simulink model "proj_parachot"  (R2015a)
settings: Solver=ode3  StartTime=0.0  StopTime=3  FixedStep=0.01  RelTol=1e-3
values from neighbouring files (symbols this model uses):
  Bj = 10    [proj_parachotM.m]
  Bp = 100    [proj_parachotM.m]
  Kr = 400    [proj_parachotM.m]
  Mj = 60    [proj_parachotM.m]
  Mp = 10    [proj_parachotM.m]
libraries: fl_lib x15, nesl_utility x7
settings Model: Creator=ahmed alaa  LastModifiedBy=ahmed alaa

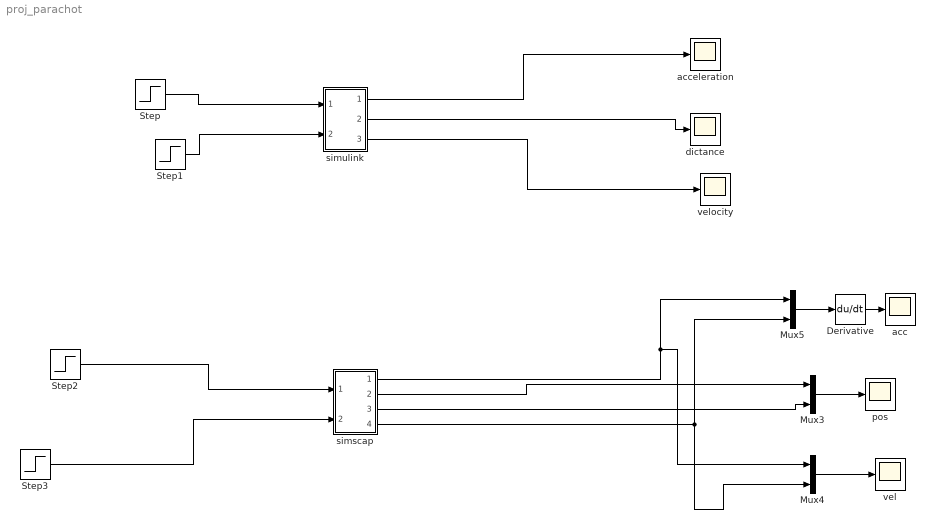
== system proj_parachot ==
  Derivative : Derivative
  Mux3 : Mux  Inputs=2
  Mux4 : Mux  Inputs=2
  Mux5 : Mux  Inputs=2
  Step{,1..3} (4 alike) : Step  Time=0  SampleTime=0
  acc : Scope
      settings: SaveName=ScopeData3
  "acceleration " : Scope
      settings: SaveName=ScopeData2
  dictance : Scope
  pos : Scope
      settings: SaveName=ScopeData4
  simscap : Subsystem
  simulink : Subsystem
  vel : Scope
      settings: SaveName=ScopeData5
  velocity : Scope
  wires:
  Step/1 -> simulink/1(In1)
  Step1/1 -> simulink/2(In2)
  simulink/1(Out1) -> "acceleration "/1
  simulink/2(Out2) -> dictance/1
  simulink/3(Out3) -> velocity/1
  simscap/3(Out3) -> Mux3/2
  simscap/2(Out2) -> Mux3/1
  Step3/1 -> simscap/2(In2)
  Step2/1 -> simscap/1(In1)
  simscap/4(Out4) -> Mux4/2, Mux5/2
  simscap/1(Out1) -> Mux5/1, Mux4/1
  Mux5/1 -> Derivative/1
  Mux3/1 -> pos/1
  Derivative/1 -> acc/1
  Mux4/1 -> vel/1

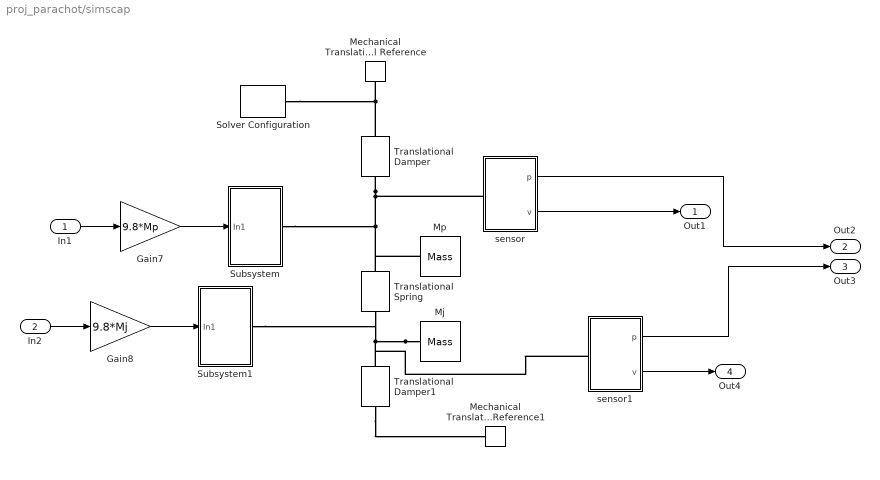
== system proj_parachot/simscap ==
  In1 : Inport
  In2 : Inport  Port=2
  Gain7 : Gain  Gain=9.8*Mp
  Gain8 : Gain  Gain=9.8*Mj
  Mechanical Translational Reference : fl_lib/Mechanical/Translational Elements/Mechanical Translational Reference
  Mechanical Translational Reference1 : fl_lib/Mechanical/Translational Elements/Mechanical Translational Reference
  Mj : fl_lib/Mechanical/Translational Elements/Mass  mass=Mj kg  v_specify=on  v_priority=High  v=20 m/s  f_specify=off  f_priority=High  f=0 N
  Mp : fl_lib/Mechanical/Translational Elements/Mass  mass=Mp kg  v_specify=on  v_priority=High  v=20 m/s  f_specify=off  f_priority=High  f=0 N
  Solver Configuration : nesl_utility/Solver Configuration  PhysicalDomain=network_engine_domain  SubClassName=solver  LeftPortType=input  RightPortType=generic  Accelerate=off  Tones=[]  Harmonics=[]  SimulateNoise=off  Profile=off  UseLocalSampling=off  EnableSwitchedLinearOptims=on  FrequencyDomain=off  UseCCode=off  RelTol=0.001  AbsTol=1e-06  MinStep=1e-09  ToWorkspace=off  RevertToSquareIcSolve=off  NumHomotopyIterations=100  DoDC=off  ResidualTolerance=1e-09  UseLocalSolver=off  LocalSolverChoice=NE_BACKWARD_EULER_ADVANCER  LocalSolverSampleTime=0.001  DoFixedCost=off  MaxNonlinIter=3  MaxModeIter=2  LinearAlgebra=Sparse  DelaysMemoryBudget=1024  AutomaticFiltering=on  FilteringTimeConstant=0.001
  Subsystem : Subsystem
  Subsystem1 : Subsystem
  Translational Damper : fl_lib/Mechanical/Translational Elements/Translational Damper  D=Bp N/(m/s)  v_specify=off  v_priority=High  v=0 m/s  f_specify=off  f_priority=High  f=0 N
  Translational Damper1 : fl_lib/Mechanical/Translational Elements/Translational Damper  D=Bj N/(m/s)  v_specify=off  v_priority=High  v=0 m/s  f_specify=off  f_priority=High  f=0 N
  Translational Spring : fl_lib/Mechanical/Translational Elements/Translational Spring  spr_rate=Kr N/m  v_specify=off  v_priority=High  v=0 m/s  f_specify=off  f_priority=High  f=0 N  x_specify=off  x_priority=High  x=0 m
  sensor : Subsystem
  sensor1 : Subsystem
  Out1 : Outport
  Out2 : Outport  Port=2
  Out3 : Outport  Port=3
  Out4 : Outport  Port=4
  wires:
  Gain7/1 -> Subsystem/1(In1)
  In2/1 -> Gain8/1
  In1/1 -> Gain7/1
  sensor1/1(p) -> Out3/1
  Gain8/1 -> Subsystem1/1(In1)
  sensor/1(p) -> Out2/1
  sensor/2(v) -> Out1/1
  sensor1/2(v) -> Out4/1
  connections:
  Translational Damper1/RConn1 -- Mechanical Translational Reference1/LConn1
  Solver Configuration/RConn1 -- Mechanical Translational Reference/LConn1 -- Translational Damper/LConn1
  Translational Damper/RConn1 -- sensor/LConn1 -- Subsystem/RConn1 -- Translational Spring/LConn1 -- Mp/LConn1
  Mj/LConn1 -- sensor1/LConn1 -- Translational Damper1/LConn1 -- Translational Spring/RConn1 -- Subsystem1/RConn1

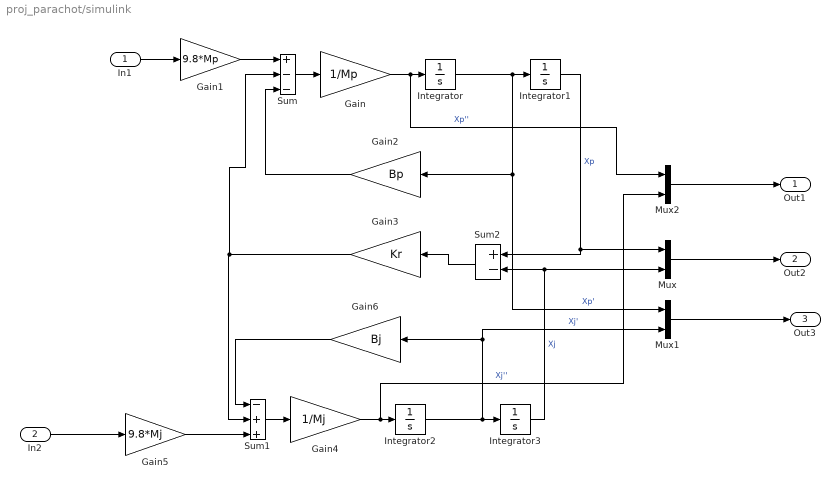
== system proj_parachot/simulink ==
  In1 : Inport
  In2 : Inport  Port=2
  Gain : Gain  Gain=1/Mp
  Gain1 : Gain  Gain=9.8*Mp
  Gain2 : Gain  Gain=Bp
  Gain3 : Gain  Gain=Kr
  Gain4 : Gain  Gain=1/Mj
  Gain5 : Gain  Gain=9.8*Mj
  Gain6 : Gain  Gain=Bj
  Integrator : Integrator  InitialCondition=20
  Integrator1 : Integrator
  Integrator2 : Integrator  InitialCondition=20
  Integrator3 : Integrator
  Mux : Mux  Inputs=2
  Mux1 : Mux  Inputs=2
  Mux2 : Mux  Inputs=2
  Sum : Sum  Inputs=+--
  Sum1 : Sum  Inputs=-++
  Sum2 : Sum  Inputs=+-
  Out1 : Outport
  Out2 : Outport  Port=2
  Out3 : Outport  Port=3
  wires:
  Sum/1 -> Gain/1
  Gain1/1 -> Sum/1
  Gain4/1 -> Mux2/2, Integrator2/1  "Xj''"
  In1/1 -> Gain1/1
  Integrator/1 -> Mux1/1, Gain2/1, Integrator1/1  "Xp'"
  Sum1/1 -> Gain4/1
  In2/1 -> Gain5/1
  Gain2/1 -> Sum/3
  Gain/1 -> Mux2/1, Integrator/1  "Xp''"
  Integrator2/1 -> Integrator3/1, Mux1/2, Gain6/1  "Xj'"
  Gain3/1 -> Sum/2, Sum1/2
  Integrator1/1 -> Mux/1, Sum2/1  "Xp"
  Mux/1 -> Out2/1
  Mux1/1 -> Out3/1
  Gain5/1 -> Sum1/3
  Integrator3/1 -> Mux/2, Sum2/2  "Xj"
  Gain6/1 -> Sum1/1
  Mux2/1 -> Out1/1
  Sum2/1 -> Gain3/1

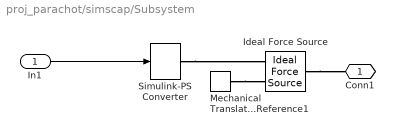
== system proj_parachot/simscap/Subsystem ==
  In1 : Inport
  Ideal Force Source : fl_lib/Mechanical/Mechanical Sources/Ideal Force Source
  Mechanical Translational Reference1 : fl_lib/Mechanical/Translational Elements/Mechanical Translational Reference
  Simulink-PS Converter : nesl_utility/Simulink-PS Converter  PhysicalDomain=network_engine_domain  SubClassName=ps_input  LeftPortType=input  RightPortType=output  PseudoPeriodic=off  Frequencies=[]  NoiseDistribution=none  NoiseParameters=[]  Unit=1  AffineConversion=off  InputFiltering=off  SimscapeFilterOrder=1  InputFilterTimeConstant=0.001  UdotUserProvided=1
  Conn1 : PMIOPort  Port=1  Side=Right
  wires:
  In1/1 -> Simulink-PS Converter/1
  connections:
  Mechanical Translational Reference1/LConn1 -- Ideal Force Source/RConn2
  Simulink-PS Converter/RConn1 -- Ideal Force Source/RConn1
  Ideal Force Source/LConn1 -- Conn1/RConn1

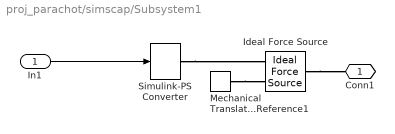
== system proj_parachot/simscap/Subsystem1 ==
  In1 : Inport
  Ideal Force Source : fl_lib/Mechanical/Mechanical Sources/Ideal Force Source
  Mechanical Translational Reference1 : fl_lib/Mechanical/Translational Elements/Mechanical Translational Reference
  Simulink-PS Converter : nesl_utility/Simulink-PS Converter  PhysicalDomain=network_engine_domain  SubClassName=ps_input  LeftPortType=input  RightPortType=output  PseudoPeriodic=off  Frequencies=[]  NoiseDistribution=none  NoiseParameters=[]  Unit=1  AffineConversion=off  InputFiltering=off  SimscapeFilterOrder=1  InputFilterTimeConstant=0.001  UdotUserProvided=1
  Conn1 : PMIOPort  Port=1  Side=Right
  wires:
  In1/1 -> Simulink-PS Converter/1
  connections:
  Ideal Force Source/LConn1 -- Conn1/RConn1
  Simulink-PS Converter/RConn1 -- Ideal Force Source/RConn1
  Mechanical Translational Reference1/LConn1 -- Ideal Force Source/RConn2

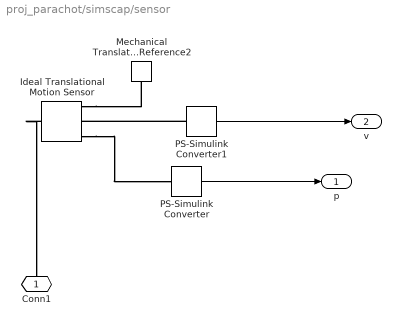
== system proj_parachot/simscap/sensor ==
  Ideal Translational Motion Sensor : fl_lib/Mechanical/Mechanical Sensors/Ideal Translational Motion Sensor  offset=0 m
  Mechanical Translational Reference2 : fl_lib/Mechanical/Translational Elements/Mechanical Translational Reference
  PS-Simulink Converter : nesl_utility/PS-Simulink Converter  PhysicalDomain=network_engine_domain  SubClassName=ps_output  LeftPortType=input  RightPortType=output  PseudoPeriodic=off  Frequencies=[]  Unit=1  AffineConversion=off
  PS-Simulink Converter1 : nesl_utility/PS-Simulink Converter  PhysicalDomain=network_engine_domain  SubClassName=ps_output  LeftPortType=input  RightPortType=output  PseudoPeriodic=off  Frequencies=[]  Unit=1  AffineConversion=off
  Conn1 : PMIOPort  Port=1  Side=Left
  p : Outport
  v : Outport  Port=2
  wires:
  PS-Simulink Converter/1 -> p/1
  PS-Simulink Converter1/1 -> v/1
  connections:
  PS-Simulink Converter1/LConn1 -- Ideal Translational Motion Sensor/RConn2
  Ideal Translational Motion Sensor/RConn3 -- PS-Simulink Converter/LConn1
  Ideal Translational Motion Sensor/RConn1 -- Mechanical Translational Reference2/LConn1
  Ideal Translational Motion Sensor/LConn1 -- Conn1/RConn1

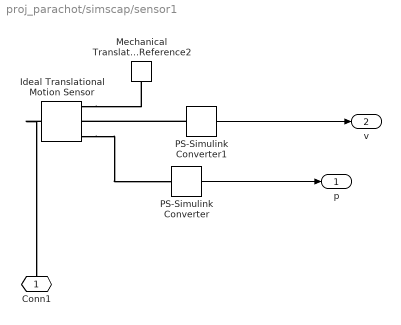
== system proj_parachot/simscap/sensor1 ==
  Ideal Translational Motion Sensor : fl_lib/Mechanical/Mechanical Sensors/Ideal Translational Motion Sensor  offset=0 m
  Mechanical Translational Reference2 : fl_lib/Mechanical/Translational Elements/Mechanical Translational Reference
  PS-Simulink Converter : nesl_utility/PS-Simulink Converter  PhysicalDomain=network_engine_domain  SubClassName=ps_output  LeftPortType=input  RightPortType=output  PseudoPeriodic=off  Frequencies=[]  Unit=1  AffineConversion=off
  PS-Simulink Converter1 : nesl_utility/PS-Simulink Converter  PhysicalDomain=network_engine_domain  SubClassName=ps_output  LeftPortType=input  RightPortType=output  PseudoPeriodic=off  Frequencies=[]  Unit=1  AffineConversion=off
  Conn1 : PMIOPort  Port=1  Side=Left
  p : Outport
  v : Outport  Port=2
  wires:
  PS-Simulink Converter1/1 -> v/1
  PS-Simulink Converter/1 -> p/1
  connections:
  Ideal Translational Motion Sensor/LConn1 -- Conn1/RConn1
  Ideal Translational Motion Sensor/RConn1 -- Mechanical Translational Reference2/LConn1
  Ideal Translational Motion Sensor/RConn3 -- PS-Simulink Converter/LConn1
  PS-Simulink Converter1/LConn1 -- Ideal Translational Motion Sensor/RConn2
